simulink model "stopwatch"  (R2018a)
settings: Solver=ode3  StartTime=0.0  StopTime=inf  FixedStep=0.1  RelTol=1e-3
libraries: MBD_blocks x7, simulink x1
settings Model: EnablePacing=on  PacingRate=1000  Creator=gerry  LastModifiedBy=leona
settings OptimizationCC: DefaultParameterBehavior=Inlined  EnhancedBackFolding=on  PassReuseOutputArgsAs=Individual arguments  OptimizeBlockOrder=speed  DifferentSizesBufferReuse=on  OptimizationCustomize=off
settings DebuggingCC: ParameterTunabilityLossMsg=error  LibraryContextMissingDiagnostic=warning
settings SFSimCC: SimUseLocalCustomCode=on  MATLABDynamicMemAlloc=off
settings RTWCC: SystemTargetFile=ert.tlc  GenCodeOnly=on  TemplateMakefile=ert_default_tmf  RTWUseLocalCustomCode=on  IncludeHyperlinkInReport=on
settings RTWCC: CustomSourceCode=|
  | #include "Buzzer.h"
  | #include "Event.h"
  | #include "WidgetConfig.h"
settings CodeAppCC: ForceParamTrailComments=on  IgnoreCustomStorageClasses=off  OperatorAnnotations=on  SimulinkDataObjDesc=on  SFDataObjDesc=on  InsertBlockDesc=on
settings ERTTargetCC: TargetLangStandard=C99 (ISO)  IncludeMdlTerminateFcn=off  SupportAbsoluteTime=off  MultiInstanceERTCode=on  CodeInterfacePackaging=Reusable function  SupportNonFinite=off  SupportComplex=off  PurelyIntegerCode=on  GenerateAllocFcn=on  InlinedParameterPlacement=NonHierarchical  ERTCustomFileTemplate=example_file_process.tlc  IndentSize=4

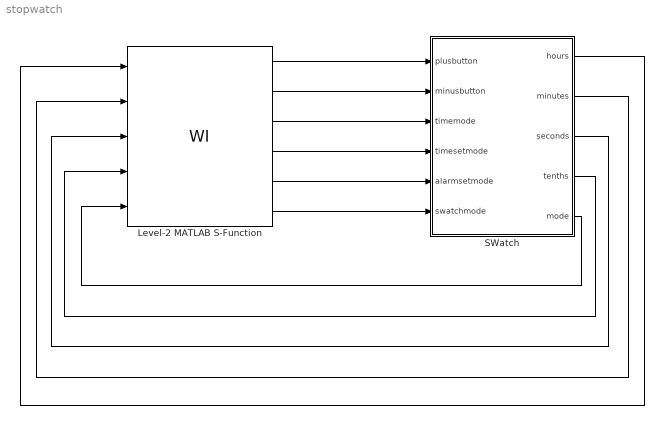
== system stopwatch ==
  Level-2 MATLAB S-Function : M-S-Function  FunctionName=WI
  SWatch : Subsystem
  wires:
  Level-2 MATLAB S-Function/1 -> SWatch/1(plusbutton)
  Level-2 MATLAB S-Function/2 -> SWatch/2(minusbutton)
  Level-2 MATLAB S-Function/3 -> SWatch/3(timemode)
  Level-2 MATLAB S-Function/4 -> SWatch/4(timesetmode)
  Level-2 MATLAB S-Function/5 -> SWatch/5(alarmsetmode)
  Level-2 MATLAB S-Function/6 -> SWatch/6(swatchmode)
  SWatch/1(hours) -> Level-2 MATLAB S-Function/1
  SWatch/2(minutes) -> Level-2 MATLAB S-Function/2
  SWatch/3(seconds) -> Level-2 MATLAB S-Function/3
  SWatch/4(tenths) -> Level-2 MATLAB S-Function/4
  SWatch/5(mode) -> Level-2 MATLAB S-Function/5

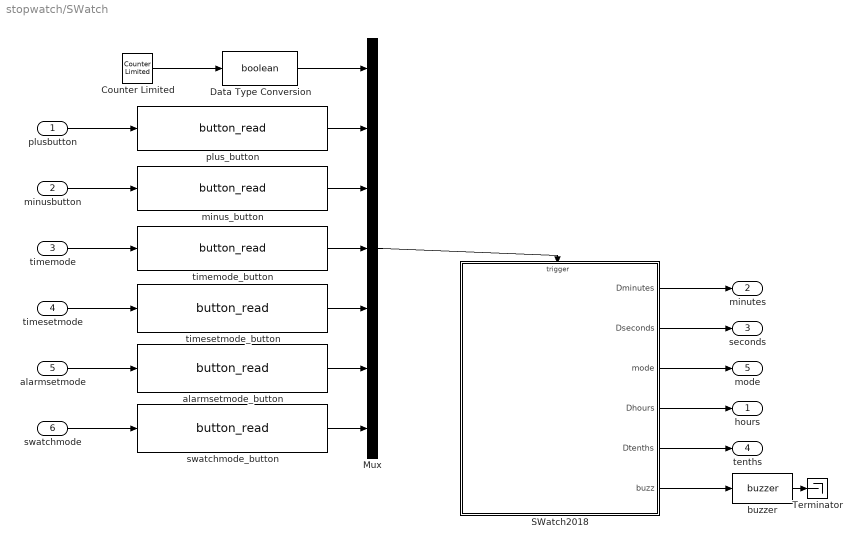
== system stopwatch/SWatch ==
  plusbutton : Inport
  minusbutton : Inport  Port=2
  timemode : Inport  Port=3
  timesetmode : Inport  Port=4
  alarmsetmode : Inport  Port=5
  swatchmode : Inport  Port=6
  Counter Limited : simulink/Sources/Counter Limited  uplimit=1  tsamp=0.1
  Data Type Conversion : DataTypeConversion  OutDataTypeStr=boolean
  Mux : Mux  Inputs=7
  SWatch2018 : Stateflow chart  TreatAsAtomicUnit=on
  Terminator : Terminator
  alarmsetmode_button : MBD_blocks/BUTTON/button_read  buttonFuncName='ALARMMODE_EV'
      settings: SourceProductName=Model Based Design ReTis
  buzzer : MBD_blocks/BUZZER/buzzer  buzzerFuncName=0
      settings: SourceProductName=Model Based Design ReTis
  minus_button : MBD_blocks/BUTTON/button_read  buttonFuncName='MINUS_EV'
      settings: SourceProductName=Model Based Design ReTis
  plus_button : MBD_blocks/BUTTON/button_read  buttonFuncName='PLUS_EV'
      settings: SourceProductName=Model Based Design ReTis
  swatchmode_button : MBD_blocks/BUTTON/button_read  buttonFuncName='SWATCHMODE_EV'
      settings: SourceProductName=Model Based Design ReTis
  timemode_button : MBD_blocks/BUTTON/button_read  buttonFuncName='TIMEMODE_EV'
      settings: SourceProductName=Model Based Design ReTis
  timesetmode_button : MBD_blocks/BUTTON/button_read  buttonFuncName='TIMESETMODE_EV'
      settings: SourceProductName=Model Based Design ReTis
  hours : Outport
  minutes : Outport  Port=2
  seconds : Outport  Port=3
  tenths : Outport  Port=4
  mode : Outport  Port=5
  wires:
  minusbutton/1 -> minus_button/1
  plusbutton/1 -> plus_button/1
  Mux/1 -> SWatch2018/Trigger
  SWatch2018/2(Dseconds) -> seconds/1
  Data Type Conversion/1 -> Mux/1
  Counter Limited/1 -> Data Type Conversion/1
  swatchmode/1 -> swatchmode_button/1
  alarmsetmode/1 -> alarmsetmode_button/1
  timesetmode/1 -> timesetmode_button/1
  SWatch2018/5(Dtenths) -> tenths/1
  SWatch2018/3(mode) -> mode/1
  SWatch2018/1(Dminutes) -> minutes/1
  SWatch2018/4(Dhours) -> hours/1
  timemode/1 -> timemode_button/1
  swatchmode_button/1 -> Mux/7
  alarmsetmode_button/1 -> Mux/6
  timemode_button/1 -> Mux/4
  timesetmode_button/1 -> Mux/5
  minus_button/1 -> Mux/3
  plus_button/1 -> Mux/2
  SWatch2018/6(buzz) -> buzzer/1
  buzzer/1 -> Terminator/1

== stateflow chart stopwatch/SWatch/SWatch2018 ==
  settings: executeAtInitialization=1
  state TimeCount [parallel]
    settings: executionOrder=2
    state Count
    (junction 143) -> (junction 140)
    (junction 145) -> (junction 143)
    (junction 148) -> (junction 145)
    (junction 140) -> Count
    (junction 110) -> (junction 148) [order 2] : {hours=hours+1}
    (junction 110) -> (junction 148) [order 1] : [hours==23]{hours=uint8(0)}
    (junction 106) -> (junction 140) [order 2] : {tenths=tenths+1}
    (junction 50) -> (junction 145) [order 2] : {minutes=minutes+1}
    (junction 45) -> (junction 143) [order 2] : {seconds=seconds+1}
    (default) -> Count : {Dtenths=uint8(0);
        | tenths=uint8(0)}
    Count -> (junction 106) : Tick
    (junction 106) -> (junction 45) [order 1] : [tenths==9]{tenths=uint8(0)}
    (junction 45) -> (junction 50) [order 1] : [seconds==59]{seconds=uint8(0)}
    (junction 50) -> (junction 110) [order 1] : [minutes==59]{minutes=uint8(0)}
  state Interface [parallel]
    en: seconds=uint8(0); minutes=uint8(0); hours=uint8(0);
    Ahours=uint8(0); Aminutes=uint8(0);
    settings: executionOrder=1
    state TimeDisplay
      en: mode=uint8(0)
      du:Dhours=hours;Dminutes=minutes;Dseconds=seconds
    state Stopwatch
      en: mode=uint8(3);
      du: Dhours=Shours; Dminutes=Sminutes;
      Dseconds=Sseconds; Dtenths=Stenths;
      state Running
      state Idle
      (default) -> Interface.Stopwatch.Idle
      Interface.Stopwatch.Idle -> Interface.Stopwatch.Running : plusbutton{send(StopwatchMgmt.stopwatchstart)}
      Interface.Stopwatch.Running -> Interface.Stopwatch.Idle : plusbutton{send(StopwatchMgmt.stopwatchpause)}
      Stopwatch -> (history) [order 1] : minusbutton{send(StopwatchMgmt.stopwatchreset)}
    state TimeSet
      en: mode=uint8(1)
      du: Dhours=hours; Dminutes=minutes; Dseconds=seconds
      (history)
      state SetHours
      state SetMinutes
      Interface.TimeSet.SetHours -> (junction 64) [order 1] : plusbutton
      Interface.TimeSet.SetMinutes -> (junction 78) [order 1] : plusbutton
      (junction 64) -> Interface.TimeSet.SetHours [order 1] : [hours==23]{hours=uint8(0)}
      (junction 78) -> Interface.TimeSet.SetMinutes [order 1] : [minutes==59]{minutes=uint8(0)}
      (junction 64) -> Interface.TimeSet.SetHours [order 2] : /{hours=hours+1}
      (junction 78) -> Interface.TimeSet.SetMinutes [order 2] : /{minutes=minutes+1}
      Interface.TimeSet.SetHours -> Interface.TimeSet.SetMinutes [order 2] : timesetmode
      (default) -> Interface.TimeSet.SetHours
      Interface.TimeSet.SetMinutes -> Interface.TimeSet.SetHours [order 3] : timesetmode
      Interface.TimeSet.SetMinutes -> (junction 137) [order 2] : minusbutton
      (junction 137) -> Interface.TimeSet.SetMinutes [order 2] : /{minutes=minutes-1}
      (junction 137) -> Interface.TimeSet.SetMinutes [order 1] : [minutes==0]{minutes=uint8(59)}
      Interface.TimeSet.SetHours -> (junction 134) [order 3] : minusbutton
      (junction 134) -> Interface.TimeSet.SetHours [order 2] : /{hours=hours-1}
      (junction 134) -> Interface.TimeSet.SetHours [order 1] : [hours==0]{hours=uint8(23)}
    state AlarmSet
      en: mode=uint8(2)
      du: Dhours=Ahours; Dminutes=Aminutes
      (history)
      state SetHours
      state SetMinutes
      Interface.AlarmSet.SetHours -> (junction 87) [order 1] : plusbutton
      Interface.AlarmSet.SetMinutes -> (junction 85) [order 1] : plusbutton
      (junction 87) -> Interface.AlarmSet.SetHours [order 1] : [Ahours==23]{Ahours=uint8(0)}
      (junction 85) -> Interface.AlarmSet.SetMinutes [order 1] : [Aminutes==59]{Aminutes=uint8(0)}
      (junction 87) -> Interface.AlarmSet.SetHours [order 2] : /{Ahours=Ahours+1}
      (junction 85) -> Interface.AlarmSet.SetMinutes [order 2] : /{Aminutes=Aminutes+1}
      (default) -> Interface.AlarmSet.SetHours
      Interface.AlarmSet.SetHours -> Interface.AlarmSet.SetMinutes [order 2] : alarmsetmode
      Interface.AlarmSet.SetMinutes -> Interface.AlarmSet.SetHours [order 3] : alarmsetmode
      Interface.AlarmSet.SetMinutes -> (junction 131) [order 2] : minusbutton
      (junction 131) -> Interface.AlarmSet.SetMinutes [order 2] : /{Aminutes=Aminutes-1}
      (junction 131) -> Interface.AlarmSet.SetMinutes [order 1] : [Aminutes==0]{Aminutes=uint8(59)}
      Interface.AlarmSet.SetHours -> (junction 123) [order 3] : minusbutton
      (junction 123) -> Interface.AlarmSet.SetHours [order 2] : /{Ahours=Ahours-1}
      (junction 123) -> Interface.AlarmSet.SetHours [order 1] : [Ahours==0]{Ahours=uint8(23)}
    Interface -> TimeDisplay [order 1] : timemode
    (default) -> TimeDisplay
    TimeDisplay -> TimeSet [order 1] : timesetmode
    TimeDisplay -> AlarmSet [order 2] : alarmsetmode
    Interface -> Stopwatch [order 2] : swatchmode
    Stopwatch -> TimeSet [order 1] : timesetmode
    Stopwatch -> AlarmSet [order 2] : alarmsetmode
    TimeSet -> AlarmSet : alarmsetmode
    AlarmSet -> TimeSet : timesetmode
  state StopwatchMgmt [parallel]
    en: Stenths = uint8(0); Sseconds = uint8(0);
    Sminutes = uint8(0); Shours = uint8(0);
    settings: executionOrder=4
    state Idle
    state Running
    (junction 182) -> (junction 183)
    (junction 184) -> (junction 182)
    (junction 167) -> (junction 184)
    (junction 183) -> StopwatchMgmt.Running
    (junction 171) -> (junction 167) [order 2] : {Shours=Shours+1}
    (junction 171) -> (junction 167) [order 1] : [Shours==23]{Shours=uint8(0)}
    (junction 176) -> (junction 183) [order 2] : {Stenths=Stenths+1}
    (junction 177) -> (junction 184) [order 2] : {Sminutes=Sminutes+1}
    (junction 170) -> (junction 182) [order 2] : {Sseconds=Sseconds+1}
    StopwatchMgmt.Idle -> StopwatchMgmt.Running : stopwatchstart
    (default) -> StopwatchMgmt.Idle
    StopwatchMgmt.Running -> StopwatchMgmt.Idle [order 1] : stopwatchpause
    StopwatchMgmt.Running -> (junction 176) [order 2] : Tick
    StopwatchMgmt -> (history) : stopwatchreset
        | {Stenths = uint8(0); Sseconds = uint8(0);
        |  Sminutes = uint8(0); Shours = uint8(0);}
    (junction 176) -> (junction 170) [order 1] : [Stenths==9]{Stenths=uint8(0)}
    (junction 170) -> (junction 177) [order 1] : [Sseconds==59]{Sseconds=uint8(0)}
    (junction 177) -> (junction 171) [order 1] : [Sminutes==59]{Sminutes=uint8(0)}
  state AlarmMgmt [parallel]
    settings: executionOrder=3
    state Silent
      en: buzz=false;
    state Buzzing
      state BuzzHigh
      state BuzzLow
      (default) -> BuzzHigh : {buzz=true}
      BuzzHigh -> BuzzLow : Tick[tenths==0]{buzz=false}
      BuzzLow -> BuzzHigh : Tick[tenths==0]{buzz=true}
    (default) -> Silent
    Silent -> Buzzing : [Ahours==hours && Aminutes==minutes && seconds==0]
    Buzzing -> Silent : [Ahours~=hours || Aminutes~=minutes || seconds>5]
  (default) -> Interface
  data: Dminutes output uint8; Dseconds output uint8; mode output uint8; Dhours output uint8; Ahours local uint8; Aminutes local uint8; hours local uint8; minutes local uint8; seconds local uint8; Dtenths output uint8; tenths local uint8; Shours local uint8; Sminutes local uint8; Sseconds local uint8; Stenths local uint8; buzz output boolean
  events: stopwatchstart local FUNCTION_CALL_EVENT; stopwatchreset local FUNCTION_CALL_EVENT; stopwatchpause local FUNCTION_CALL_EVENT; Tick input EITHER_EDGE_EVENT; plusbutton input RISING_EDGE_EVENT; minusbutton input RISING_EDGE_EVENT; timemode input RISING_EDGE_EVENT; timesetmode input RISING_EDGE_EVENT; alarmsetmode input RISING_EDGE_EVENT; swatchmode input RISING_EDGE_EVENT
